simulink model "buck_observer"  (R2020a)
settings: Solver=VariableStepAuto  StartTime=0.0  StopTime=0.1  MaxStep=1e-6
undefined symbols (not defined in the file): DiscIntNeverNeededParam
libraries: powerlib x11, eeGeneralControl x2, eeLuenbergerObserver x1, powerlib_meascontrol x1
settings Model: Creator=Slash  LastModifiedBy=Slash
settings SolverCC: AutoInsertRateTranBlk=on

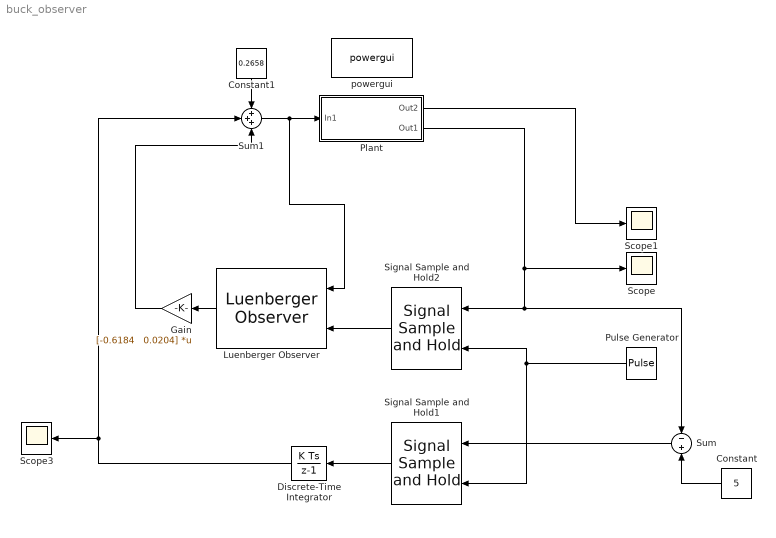
== system buck_observer ==
  Constant : Constant  Value=5
  Constant1 : Constant  Value=0.2658
  Discrete-Time Integrator : DiscreteIntegrator  gainval=1.5  SampleTime=0.001  ICPrevOutput=DiscIntNeverNeededParam  ICPrevScaledInput=DiscIntNeverNeededParam
  Gain : Gain  Gain="[-0.6184   0.0204]"  Multiplication=Matrix(K*u)
  Luenberger Observer : eeLuenbergerObserver/Luenberger Observer  StateSpaceType=Discrete-time  Ad=[0.2113,-0.0605;10.7447,0.1815]  Bd=[1.0168; 10.5637]  Cd=[0,1]  Dd=0  A=1  B=1  C=1  D=1  ObserverDesign=Desired eigenvalues  Ld=1  DesiredEigenvalues=[0.1,0.11]  x0=[0,0]  Tsd=0.1  Ts=0.001
      settings: SourceProductBaseCode=PS
  Plant : Subsystem
  Pulse Generator : DiscretePulseGenerator  PulseType=Time based  Period=0.001
  Scope : Scope
  Scope1 : Scope
  Scope3 : Scope
  Signal Sample and Hold1 : eeGeneralControl/Signal Sample and Hold  LabelModeActiveChoice=Discrete  x0=0  Ts=0.001
      settings: SourceProductBaseCode=PS
  Signal Sample and Hold2 : eeGeneralControl/Signal Sample and Hold  LabelModeActiveChoice=Discrete  x0=0  Ts=0.001
      settings: SourceProductBaseCode=PS
  Sum : Sum  Inputs=-+
  Sum1 : Sum  Inputs=+++
  powergui : powerlib/powergui  Priority=1  SimulationMode=Continuous  SampleTime=50e-6  frequency=60  Iterations=50  frequencyindice=0  Pbase=100e6  ErrMax=1e-4  UnitsV=kV  UnitsW=MW  buscounter=0  FunctionMessages=off  echomessages=off  EnableUseOfTLC=off  CurrentSourceSwitches=off  DisableSnubberDevices=off  DisableRonSwitches=off  DisableVfSwitches=off  DisplayEquations=off  AutomaticDiscreteSolvers=off  SolverType=Tustin/Backward Euler (TBE)  Interpol=off  ExternalGateDelay=off  methode=off  Ts=100  x0status=blocks  SPID=on  SwTol=0  HookPort=off  NonlinearTolerance=1e-4  nMaxIteration=100  ContinueOnMaxIteration=off  RestoreLinks=warning  ResistiveCurrentMeasurement=off  Frange=[0:2:500]  Ylog=off  Xlog=on  ShowGrid=off  save=off  variable=ZData  structure=0  ZoomFFT=off  StartTime=0.0  cycles=1  DisplayStyle=1  fundamental=60  FreqAxis=off  MaxFrequency=1000  frequencyindicesteady=1  RmsSteady=1  display=off
  wires:
  Constant/1 -> Sum/2
  Plant/1(Out2) -> Scope1/1
  Sum1/1 -> Luenberger Observer/1, Plant/1(In1)
  Constant1/1 -> Sum1/1
  Pulse Generator/1 -> Signal Sample and Hold1/2, Signal Sample and Hold2/2
  Plant/2(Out1) -> Sum/1, Signal Sample and Hold2/1, Scope/1
  Signal Sample and Hold1/1 -> Discrete-Time Integrator/1
  Gain/1 -> Sum1/3
  Discrete-Time Integrator/1 -> Scope3/1, Sum1/2
  Sum/1 -> Signal Sample and Hold1/1
  Signal Sample and Hold2/1 -> Luenberger Observer/2
  Luenberger Observer/1 -> Gain/1

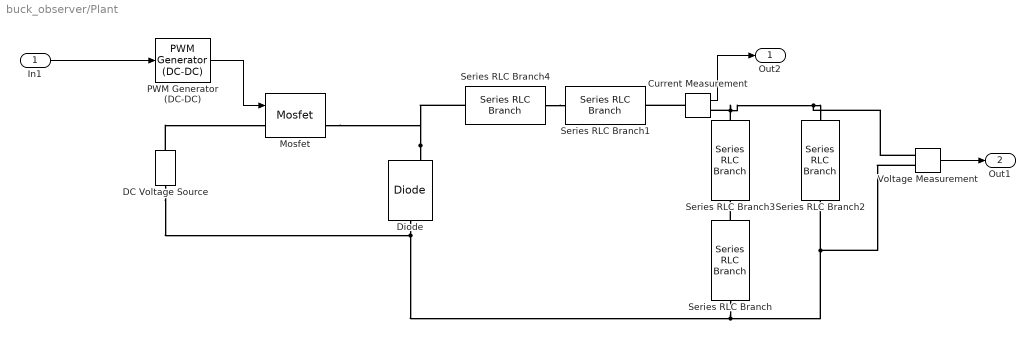
== system buck_observer/Plant ==
  In1 : Inport
  Current Measurement : powerlib/Measurements/Current Measurement  PhasorSimulation=off  OutputType=Complex  PSBequivalent=0
  DC Voltage Source : powerlib/Electrical Sources/DC Voltage Source  Amplitude=15  Measurements=None
  Diode : powerlib/Power Electronics/Diode  Ron=0.001  Lon=0  Vf=0.1  IC=0  UseSnubber=0  Rs=500  Cs=250e-9  Measurements=on
  Mosfet : powerlib/Power Electronics/Mosfet  Ron=0.05  Lon=0  Rd=0.01  Vfd=0  IC=0  Rs=1e5  Cs=inf  Measurements=on
  PWM Generator (DC-DC) : powerlib_meascontrol/Pulse & Signal Generators/PWM Generator (DC-DC)  Fsw=20000  Ts=0
  Series RLC Branch : powerlib/Elements/Series RLC Branch  LConnTagsString=__new0  RConnTagsString=__new0  BranchType=C  Resistance=1  Inductance=1e-3  SetiL0=off  InitialCurrent=0  Capacitance=56e-6  Setx0=off  InitialVoltage=0  Measurements=None
  Series RLC Branch1 : powerlib/Elements/Series RLC Branch  LConnTagsString=__new0  RConnTagsString=__new0  BranchType=L  Resistance=1  Inductance=10e-3  SetiL0=off  InitialCurrent=0  Capacitance=1e-6  Setx0=off  InitialVoltage=0  Measurements=None
  Series RLC Branch2 : powerlib/Elements/Series RLC Branch  LConnTagsString=__new0  RConnTagsString=__new0  BranchType=R  Resistance=100  Inductance=1e-3  SetiL0=off  InitialCurrent=0  Capacitance=1e-6  Setx0=off  InitialVoltage=0  Measurements=None
  Series RLC Branch3 : powerlib/Elements/Series RLC Branch  LConnTagsString=__new0  RConnTagsString=__new0  BranchType=R  Resistance=0.33  Inductance=1e-3  SetiL0=off  InitialCurrent=0  Capacitance=1e-6  Setx0=off  InitialVoltage=0  Measurements=None
  Series RLC Branch4 : powerlib/Elements/Series RLC Branch  LConnTagsString=__new0  RConnTagsString=__new0  BranchType=R  Resistance=1.6  Inductance=1e-3  SetiL0=off  InitialCurrent=0  Capacitance=1e-6  Setx0=off  InitialVoltage=0  Measurements=None
  Voltage Measurement : powerlib/Measurements/Voltage Measurement  PhasorSimulation=off  OutputType=Complex  PSBequivalent=0
  Out2 : Outport
  Out1 : Outport  Port=2
  wires:
  Voltage Measurement/1 -> Out1/1
  PWM Generator (DC-DC)/1 -> Mosfet/1
  In1/1 -> PWM Generator (DC-DC)/1
  Current Measurement/1 -> Out2/1
  connections:
  Diode/LConn1 -- DC Voltage Source/LConn1 -- Voltage Measurement/LConn2 -- Series RLC Branch2/RConn1 -- Series RLC Branch/RConn1
  Diode/RConn1 -- Series RLC Branch4/RConn1 -- Mosfet/RConn1
  Series RLC Branch3/LConn1 -- Current Measurement/RConn1 -- Series RLC Branch2/LConn1 -- Voltage Measurement/LConn1
  Series RLC Branch/LConn1 -- Series RLC Branch3/RConn1
  DC Voltage Source/RConn1 -- Mosfet/LConn1
  Series RLC Branch4/LConn1 -- Series RLC Branch1/LConn1
  Current Measurement/LConn1 -- Series RLC Branch1/RConn1
